simulink model "ECU_model"  (Simulink 8.8)
settings: Solver=VariableStepAuto  StartTime=0.0  StopTime=10.0  RelTol=1e-3  EnableMultiTasking=on
libraries: MFMdl1 x1, MFMdl2 x1, MFMdl3 x1, MFMdl4 x1, MFMdl5 x1, MFMdl6 x1, MFMdl7 x1, MFMdl8 x1
settings Model: Creator=The MathWorks, Inc.  LastModifiedBy=viett
settings DataIOCC: SaveFormat=Dataset  SignalLoggingSaveFormat=Dataset
settings DebuggingCC: UnderspecifiedInitializationDetection=Simplified  MergeDetectMultiDrivingBlocksExec=error  FcnCallInpInsideContextMsg=error  AllowSymbolicDim=off  StateNameClashWarn=none
settings HardwareCC: ProdBitPerPointer=64  ProdBitPerSizeT=64  ProdBitPerPtrDiffT=64  ProdLargestAtomicFloat=Float  ProdIntDivRoundTo=Zero  ProdEndianess=LittleEndian  ProdWordSize=64  ProdHWDeviceType=Intel->x86-64 (Windows64)
settings GRTTargetCC: GeneratePreprocessorConditionals=Use local settings  CombineOutputUpdateFcns=on  GRTInterface=off

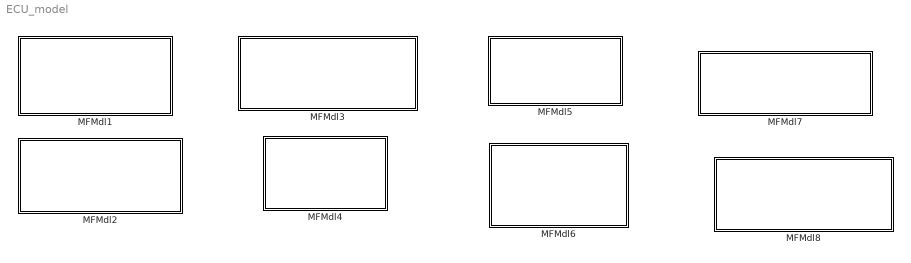
== system ECU_model ==
  MFMdl1 : Subsystem
  MFMdl2 : Subsystem
  MFMdl3 : Subsystem
  MFMdl4 : Subsystem
  MFMdl5 : Subsystem
  MFMdl6 : Subsystem
  MFMdl7 : Subsystem
  MFMdl8 : Subsystem

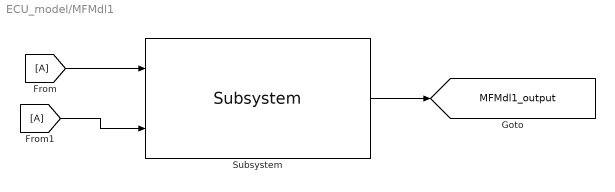
== system ECU_model/MFMdl1 ==
  Subsystem : MFMdl1/Subsystem
  tag scope: MFMdl1_output=global
  wires:
  Subsystem/1 -> [MFMdl1_output]
  [A] -> Subsystem/1
  [A] -> Subsystem/2

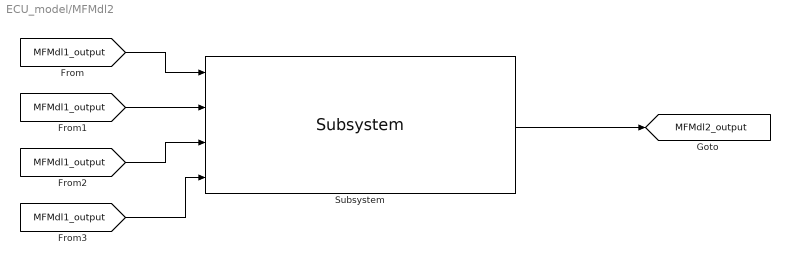
== system ECU_model/MFMdl2 ==
  Subsystem : MFMdl2/Subsystem
  tag scope: MFMdl2_output=global
  wires:
  Subsystem/1 -> [MFMdl2_output]
  [MFMdl1_output] -> Subsystem/1
  [MFMdl1_output] -> Subsystem/2
  [MFMdl1_output] -> Subsystem/3
  [MFMdl1_output] -> Subsystem/4

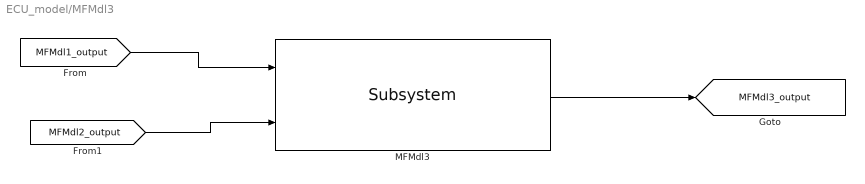
== system ECU_model/MFMdl3 ==
  MFMdl3 : MFMdl3/Subsystem
  tag scope: MFMdl3_output=global
  wires:
  MFMdl3/1 -> [MFMdl3_output]
  [MFMdl1_output] -> MFMdl3/1
  [MFMdl2_output] -> MFMdl3/2

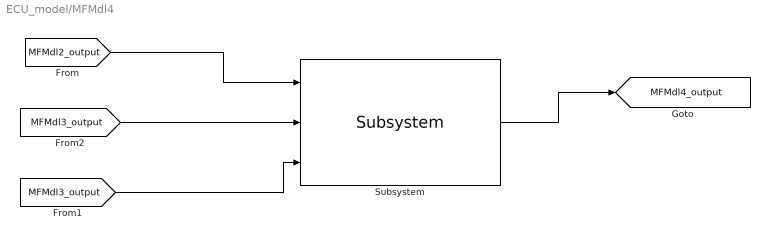
== system ECU_model/MFMdl4 ==
  Subsystem : MFMdl4/Subsystem
  tag scope: MFMdl4_output=global
  wires:
  Subsystem/1 -> [MFMdl4_output]
  [MFMdl2_output] -> Subsystem/1
  [MFMdl3_output] -> Subsystem/2
  [MFMdl3_output] -> Subsystem/3

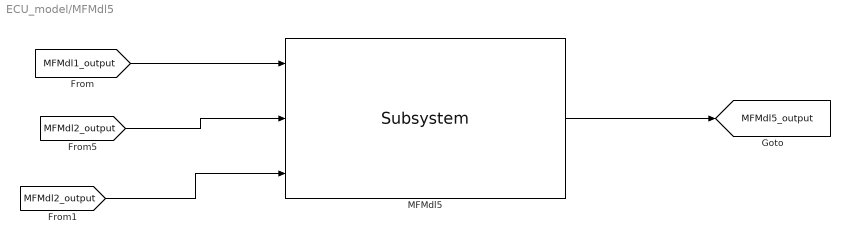
== system ECU_model/MFMdl5 ==
  MFMdl5 : MFMdl5/Subsystem
  tag scope: MFMdl5_output=global
  wires:
  MFMdl5/1 -> [MFMdl5_output]
  [MFMdl1_output] -> MFMdl5/1
  [MFMdl2_output] -> MFMdl5/2
  [MFMdl2_output] -> MFMdl5/3

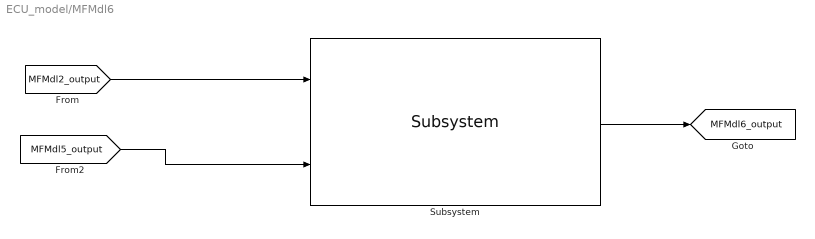
== system ECU_model/MFMdl6 ==
  Subsystem : MFMdl6/Subsystem
  tag scope: MFMdl6_output=global
  wires:
  Subsystem/1 -> [MFMdl6_output]
  [MFMdl2_output] -> Subsystem/1
  [MFMdl5_output] -> Subsystem/2

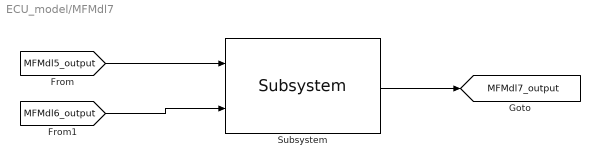
== system ECU_model/MFMdl7 ==
  Subsystem : MFMdl7/Subsystem
  tag scope: MFMdl7_output=global
  wires:
  [MFMdl5_output] -> Subsystem/1
  [MFMdl6_output] -> Subsystem/2
  Subsystem/1 -> [MFMdl7_output]

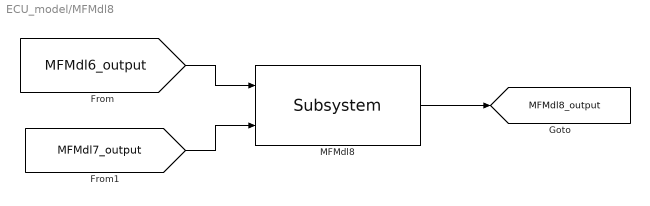
== system ECU_model/MFMdl8 ==
  MFMdl8 : MFMdl8/Subsystem
  tag scope: MFMdl8_output=global
  wires:
  [MFMdl6_output] -> MFMdl8/1
  [MFMdl7_output] -> MFMdl8/2
  MFMdl8/1 -> [MFMdl8_output]
